simulink model "simpowered_stepper_drive"  (R2013b)
settings: Solver=ode23t  StartTime=0.0  StopTime=0.25  FixedStep=Ts  MaxStep=2e-5
PreLoadFcn:
  | assignin('base','Ts',1e-6);
undefined symbols (not defined in the file): Ts
libraries: powerlib x4
Description:
  | Copyright 2008-2013 The MathWorks, Inc.
settings Model: ExtModeAutoUpdateStatusClock=off  Creator=MathWorks  LastModifiedBy=snikitin
settings DataIOCC: SignalLoggingSaveFormat=ModelDataLogs
settings OptimizationCC: ExpressionDepthLimit=2147483647  InitFltsAndDblsToZero=on
settings DebuggingCC: SignalResolutionControl=TryResolveAllWithWarning  FcnCallInpInsideContextMsg=UseLocalSettings  StateNameClashWarn=warning
settings GRTTargetCC: CombineOutputUpdateFcns=off  GRTInterface=on

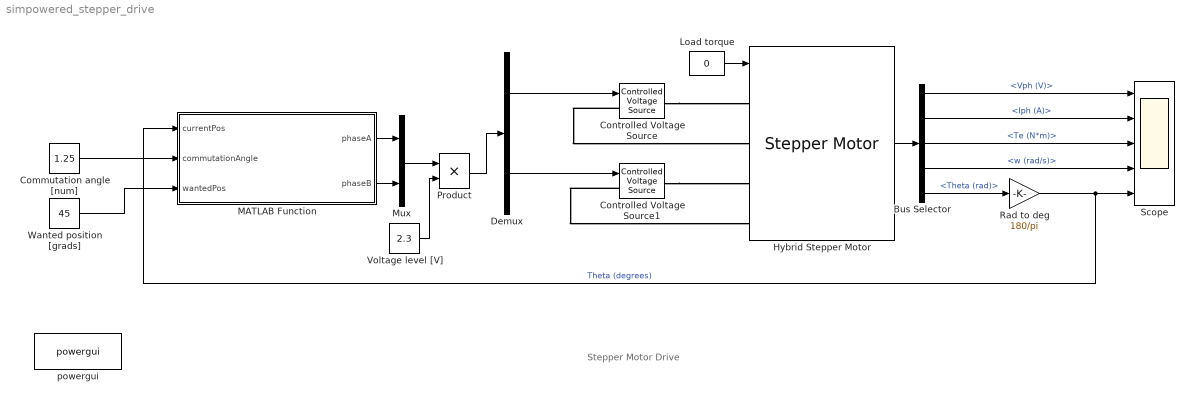
== system simpowered_stepper_drive ==
  note: Stepper Motor Drive
  Bus Selector : BusSelector  OutputSignals=Vph (V),Iph (A),Te (N*m),w (rad/s),Theta (rad)
  Commutation angle [num] : Constant  Value=1.25
  Controlled Voltage Source : powerlib/Electrical Sources/Controlled Voltage Source  Initialize=on  Source_Type=AC  Amplitude=0  Phase=0  Frequency=0  Measurements=None
  Controlled Voltage Source1 : powerlib/Electrical Sources/Controlled Voltage Source  Initialize=on  Source_Type=AC  Amplitude=0  Phase=0  Frequency=0  Measurements=None
  Demux : Demux  Outputs=2
  Hybrid Stepper Motor : powerlib/Machines/Stepper Motor  MotorType=Permanent-magnet / Hybrid  NumberOfPhases_1=2  NumberOfPhases_2=3  PresetModel_1=<empty>  PresetModel_2=<empty>  L=1.65e-3  Lmax=10e-3  Lmin=2e-3  R=0.77  Step_angle=1.8  Psim=0.00853  Tdm=0.001  J=2.8e-05  B=1e-7*1000  w0=0  pos0=0  TsPowergui=0  TsBlock=-1
  Load torque : Constant  Value=0
  MATLAB Function : MATLAB Function  TreatAsAtomicUnit=on
  Mux : Mux  Inputs=2
  Product : Product
  Rad to deg : Gain  Gain=180/pi
  Scope : Scope  NumInputPorts=5
      settings: TimeRange=0.25  YMin=-35~-3~-0.35~-1~0  YMax=35~3~0.25~9~60  SaveName=VIX
  Voltage level [V] : Constant  Value=2.3
  Wanted position [grads] : Constant  Value=45
  powergui : powerlib/powergui  SimulationMode=Discrete  SolverType=Tustin  SampleTime=Ts  frequency=60  SPID=off  DisableSnubberDevices=off  DisableRonSwitches=off  DisableVfSwitches=off  SwTol=0  Interpol=off  DisplayEquations=off  frequencyindice=0  Pbase=100e6  ErrMax=1e-4  Iterations=50  UnitsV=kV  UnitsW=MW  FunctionMessages=off  echomessages=off  HookPort=off  EnableUseOfTLC=off  x0status=blocks  RestoreLinks=warning  ResistiveCurrentMeasurement=off  Frange=[0:2:500]  Ylog=off  Xlog=on  ShowGrid=off  save=off  variable=ZData  ZoomFFT=on  StartTime=0.0  cycles=1  DisplayStyle=1  fundamental=60  FreqAxis=off  MaxFrequency=1000  frequencyindicesteady=1  RmsSteady=1  display=off  Ts=0  methode=off
  wires:
  Load torque/1 -> Hybrid Stepper Motor/1
  Hybrid Stepper Motor/1 -> Bus Selector/1
  Bus Selector/1 -> Scope/1  "<Vph (V)>"
  Bus Selector/2 -> Scope/2  "<Iph (A)>"
  Bus Selector/3 -> Scope/3  "<Te (N*m)>"
  Bus Selector/4 -> Scope/4  "<w (rad/s)>"
  Rad to deg/1 -> MATLAB Function/1(currentPos), Scope/5  "Theta (degrees)"
  Bus Selector/5 -> Rad to deg/1  "<Theta (rad)>"
  MATLAB Function/1(phaseA) -> Mux/1
  MATLAB Function/2(phaseB) -> Mux/2
  Wanted position [grads]/1 -> MATLAB Function/3(wantedPos)
  Commutation angle [num]/1 -> MATLAB Function/2(commutationAngle)
  Voltage level [V]/1 -> Product/2
  Mux/1 -> Product/1
  Demux/2 -> Controlled Voltage Source1/1
  Demux/1 -> Controlled Voltage Source/1
  Product/1 -> Demux/1
  connections:
  Controlled Voltage Source/LConn1 -- Hybrid Stepper Motor/LConn2
  Controlled Voltage Source/RConn1 -- Hybrid Stepper Motor/LConn1
  Controlled Voltage Source1/RConn1 -- Hybrid Stepper Motor/LConn3
  Controlled Voltage Source1/LConn1 -- Hybrid Stepper Motor/LConn4

== matlab function simpowered_stepper_drive/MATLAB Function ==
  data: currentPos input; commutationAngle input; wantedPos input; phaseA output; phaseB output
function [phaseA, phaseB] = setVoltage(currentPos, commutationAngle, wantedPos)
    persistent initialized;
    persistent lastPhaseA;
    persistent lastPhaseB;
    persistent direction;
    persistent lastActivatedState;
    
    if isempty(initialized)
        lastPhaseA  = 0;
        lastPhaseB  = 0;
        initialized = 1;
        direction   = sign(wantedPos);
        lastActivatedState = nan;
    end

    if (wantedPos - currentPos)*direction <= 0
        phaseA = 0;
        phaseB = 0;
        
        return
    end

    nextPhasesState = calculateNextPhasesState(currentPos, direction, commutationAngle);

    if lastActivatedState ~= nextPhasesState
        [lastPhaseA, lastPhaseB] = setWindingSignals(nextPhasesState);
        lastActivatedState = nextPhasesState;
    end

    phaseA = lastPhaseA;
    phaseB = lastPhaseB;
end

function nextPhasesState = calculateNextPhasesState(currentPosition, direction, commutationAngle) 
    ROTOR_STEP          = 1.8;
    NUMBER_OF_STATES    = 4;
    nextState     = nan;
    
    fuzzyAbsStepNumber          = currentPosition / ROTOR_STEP;
        
    if direction > 0 
        nextState = floor(fuzzyAbsStepNumber + commutationAngle);
    else
        nextState = ceil(fuzzyAbsStepNumber - commutationAngle);
    end
 
    nextPhasesState = mod(nextState, NUMBER_OF_STATES);
end

function [phaseA, phaseB] = setWindingSignals(newState)
    DISABLED            = 0;
    NORMAL_POLARITY     = 1;
    INVERTED_POLARITY   = -1;

    if newState == 0
        phaseA = NORMAL_POLARITY;
        phaseB = DISABLED;

    elseif newState == 1
        phaseA = DISABLED;
        phaseB = NORMAL_POLARITY;

    elseif newState == 2
        phaseA = INVERTED_POLARITY;
        phaseB = DISABLED;

    elseif newState == 3
        phaseA = DISABLED;
        phaseB = INVERTED_POLARITY;

    else
        phaseA = DISABLED;
        phaseB = DISABLED;
        disp('Wrong state recieved')
    end
end
